simulink library "Valeo_Simulink_Library_EC"  (R2020b)
settings: Solver=ode45  StartTime=0.0  StopTime=10.0  RelTol=1e-3  EnableMultiTasking=on
undefined symbols (not defined in the file): A, B, C, Count_Max, D, InitValue, j, ke, kf, kt, L, Length, MaxIniVal, MaxVal, MinVal, NumBits1, NumBits2, P, p0, Q, R, Simulink_Library, Ts, x0
libraries: $bdroot x9, simulink x4, fixpt_dtprop x4
(part 1 of 4)
Description:
  | This is based on VSL V5.1.0
settings Model: Creator=KROS  LastModifiedBy=mchawa
settings DataIOCC: LimitDataPoints=on  SaveFormat=Array  SignalLoggingSaveFormat=ModelDataLogs  ReturnWorkspaceOutputs=off
settings OptimizationCC: ExpressionDepthLimit=2147483647  LifeSpan=inf
settings DebuggingCC: UnderspecifiedInitializationDetection=Classic  MergeDetectMultiDrivingBlocksExec=none  SolverPrmCheckMsg=warning  MultiTaskDSMMsg=warning  MultiTaskCondExecSysMsg=none  StateNameClashWarn=warning  SFUnexpectedBacktrackingDiag=warning  SFNoUnconditionalDefaultTransitionDiag=warning  SFExecutionAtInitializationDiag=none  ArithmeticOperatorsInVariantConditions=warning
settings HardwareCC: ProdBitPerPointer=32  ProdBitPerSizeT=32  ProdBitPerPtrDiffT=32  ProdLargestAtomicFloat=None  ProdIntDivRoundTo=Undefined  ProdEndianess=Unspecified  ProdWordSize=32  ProdHWDeviceType=32-bit Generic
settings ModelReferenceCC: PropagateSignalLabelsOutOfModel=off
settings SFSimCC: SimUseLocalCustomCode=off  CustomCodeUndefinedFunction=UseInterfaceOnly
settings RTWCC: RTWUseLocalCustomCode=off
settings CodeAppCC: StateflowObjectComments=on
settings GRTTargetCC: TargetLangStandard=C89/C90 (ANSI)
settings ConfigComp: CovMetricSettings=dw  CovSaveCumulativeToWorkspaceVar=on  CovSaveSingleToWorkspaceVar=on  CovExternalEMLEnable=off

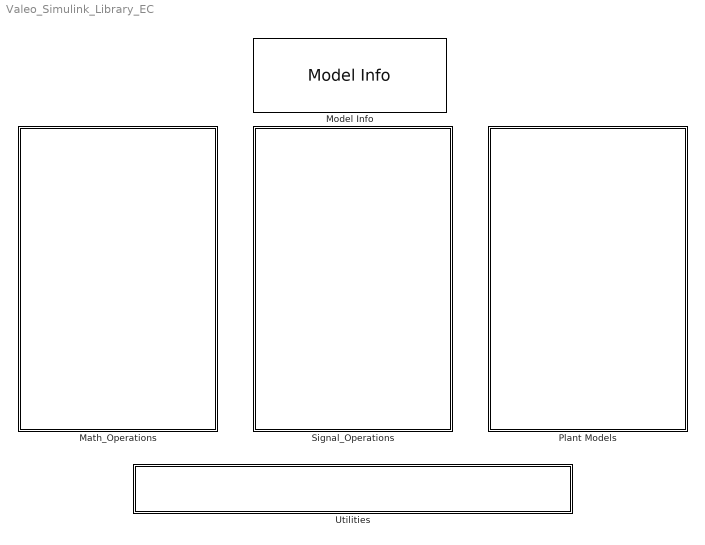
== system Valeo_Simulink_Library_EC ==
  Math_Operations : Subsystem  Description=Math Operations
  Model Info : simulink/Model-Wide Utilities/Model Info  Frame=on  DisplayStringWithTags=|  HorizontalTextAlignment=Left  LeftAlignmentValue=0.02
      | Model Info
      | 
      | Name: %<ModelName>
      | 
      | Description: %<Description>
  Plant Models : Subsystem
  Signal_Operations : Subsystem  Description=Signal Operations
  Utilities : Subsystem  Description=Utilities

== system Valeo_Simulink_Library_EC/Math_Operations ==
  Barycentre : Subsystem  RequirementInfo={} %GIDa_964ea1e7_ae9e_4180_bee1_c2dc4593188a  mask(VSL_Barycentre){}
      mask help:
      | The block 'VSL_Barycentre' calculates the weighted average or centroid of 2 variables 'In1' and 'In2'.
      |
      | Out= In1*Rate+(1-Rate)*In2
      | with 'Rate' value between 0 and 1.
      |
      | In1, In2, Rate et Out must have the same DataType
      | Inputs:
      | - 'In1': fist input for calculation
      | - 'In2': second input for calculation
      | - 'Rate': normalized weight cofficient between 0 and 1
      |
      | Output:
      | - 'Out': centroid value
      mask Help:
      | The block 'VSL_Barycentre' calculates the weighted average or centroid of 2 variables 'In1' and 'In2'.
      | 
      | Out= In1*Rate+(1-Rate)*In2
      | with 'Rate' value between 0 and 1.
      | If 'Rate'>1, 'Rate'=1.
      | If 'Rate'<0, 'Rate'=1.
      | 
      | In1, In2, Rate et Out must have the same DataType
      | Inputs:
      | - 'In1': fist input for calculation
      | - 'In2': second input for calculation
      | - 'Rate': weight cofficient between 0 and 1
      | 
      | Output:
      | - 'Out': weighted average value or centroid
      mask Display:
      | plot([0.3 0.7],[0.4 0.4])
      | plot([0.3 0.5 0.7],[0.4 0.8 0.4])
      | plot([0.3 0.8],[0.4 0.7])
      | plot([0.2 0.7],[0.7 0.4])
      | plot([0.5 0.5],[0.8 0.25])
      | text(0.45,0.59,'G');
      | patch([0.88 0.93 0.94 0.99 0.98 0.94 0.9 0.88], [0.11 0.01 0.01 0.11 0.11 0.026 0.11 0.11], [0 1 0])
  CountdownTimer : Subsystem  Description=CountdownTimer  RequirementInfo={} %GIDa_33143a65_bd33_4657_a3cb_95dcb456cb04  mask(VSL_CountdownTimer){MaxIniVal=MaxIniVal}
      mask prompts: MaxIniVal "Maximum Initial Value:"
      mask help:
      | The 'VSL_CountdownTimer' block performs a countdown from 'IniVal' value (in second), with 'Dec' decrement at each step ('Dec' in second too).
      | A pulse on input 'Strt' launches the countdown.
      | The 'VSL_CountdownTimer' could be reset to 0 if input 'Rst' is set to 1.
      | Reset has higher priority than 'Strt', so nothing happen when 'Rst' is set to 1.
      |
      | The parameter 'MaxIniVal' allows to set the maximum threshold to the initial value.
      |
      | The output 'Out' indicates the countdown status (1 active , 0 inactive) .
      | The counter value 'Val' indicates the remaining time to reach 0 value.
      |
      | The inputs 'Strt' and 'Rst', and the output 'Out' are 'boolean'.
      | 'IniVal', 'Dec', 'Val' are scalars.
      |
      | This block can be used with a variable decrement 'Dec', but the duration ('IniVal') is fixed when it is launched.
      |
      | Inputs:
      | - 'Strt': boolean command with a pulse to launch the countdown
      | - 'Rst': boolean to reset the counter to 0 (all outputs are set to 0 when is equal to 1)
      | - 'IniVal': initial value of duration of the countdown (in second)
      | - 'Dec': sample time (can vary during countdown execution) (in second)
      |
      | Outputs:
      | - 'Out': boolean that indicates the countdown status (1 active , 0 inactive)
      | - 'Val': indicates the remaining time to reach 0 value.
      |
      | Parameter:
      | - 'MaxIniVal': maximum value of the initial value (saturation) (in second)
      settings: AttributesFormatString=MaxIniVal=%<MaxIniVal>
      mask Help:
      | The 'VSL_CountdownTimer' block performs a countdown from 'IniVal' value (in second), with 'Dec' decrement at each step ('Dec' in second too).
      | A pulse on input 'Strt' launches the countdown.
      | The 'CountdownTimer' could be reset to 0 if input 'Rst' is set to 1.
      | Reset has higher priority than 'Strt', so nothing happen when 'Rst' is set to 1.
      | 
      | The parameter 'MaxIniVal' allows to set the maximum threshold to the initial value.
      | 
      | The output 'Out' indicates the countdown status (1 active , 0 inactive) .
      | The counter value 'Val' indicates the remaining time to reach 0 value.
      | 
      | The inputs 'Strt' and 'Rst', and the output 'Out' are 'boolean'.
      | 'IniVal', 'Dec', 'Val' are scalars.
      | 
      | This block can be used with a variable decrement 'Dec', but the duration ('IniVal') is fixed when it is launched.
      | 
      | Inputs:
      | - 'Strt': boolean command with a pulse to launch the countdown
      | - 'Rst': boolean to reset the counter to 0 (all outputs are set to 0 when is equal to 1)
      | - 'IniVal': initial value of duration of the countdown (in second)
      | - 'Dec': sample time (can vary during countdown execution) (in second)
      | 
      | Outputs:
      | - 'Out': boolean that indicates the countdown status (1 active , 0 inactive)
      | - 'Val': indicates the remaining time to reach 0 value.
      | 
      | Parameter:
      | - 'MaxIniVal': maximum value of the initial value (saturation) (in second)
      mask Display:
      | plot(0,0,100,100,[80,70,40,40,30],[20,20,80,20,20])
      | patch(100*[0.88 0.93 0.94 0.99 0.98 0.94 0.9 0.88], 100*[0.11 0.01 0.01 0.11 0.11 0.026 0.11 0.11], [0 1 0])
  Counter : Subsystem  RequirementInfo={} %GIDa_ad99af80_5a44_4606_b9f7_25513ebf5aeb  mask(VSL_Counter){Inc_parm=on, maxFlag=off, Reset_flag=on, InitialFlag=off, MaxCntFlag=off, Cnt_Max=Count_Max}
      mask prompts: Inc_parm "Enable Inc"; maxFlag "Enable MaxFlag"; Reset_flag "Enable Rst"; InitialFlag "Enable InitialVal"; MaxCntFlag "Enable Count_Max"; Cnt_Max "Enter Maximum Value of the Counter"
      mask help:
      | The "VSL_Counter" block increments a counter of the value Inc at each time step if Inc set as a input else counter increment by one when it is activated (Ena = 1). The Cnt output is frozen when the block is deactivated and reset to InitialVal thanks to the "Rst" input (Rst = 1).
      |
      | The Inc and Cnt data are expressed in the same unit, if Inc is expressed in seconds then Cnt is also expressed in seconds.
      |
      | About all inports
      | ------------------------
      | =>  'Inc' is the value of the counter increment per each sample.
      | =>  'Rst' (Boolean) reset the counter (counter start counting from zero if Rst =1).
      | =>  'Ena' (boolean) allows to activate the counter if Ena = 1 else  Deactivate .
      | =>  'InitialVal' can take intial value of the counter for the first sample.
      | =>  'Count_Max'  is a value to count the counter upto this maximum value.
      |
      | About all outports
      | ------------------------
      | => 'Cnt' is counting value of the counter it can update each sample time
      | => 'MaxFlag' (boolean) it is a flag indicates counter reached to Count_Max
      mask init:
      | ValeoSimulinkLibrary.Counter_MaxFlag(gcb);
      | ValeoSimulinkLibrary.Counter_reset(gcb);
      | ValeoSimulinkLibrary.Counter_Inc(gcb);
      | ValeoSimulinkLibrary.Counter_InitialVal(gcb);
      | ValeoSimulinkLibrary.Counter_MaxCount(gcb);
      mask Help:
      | The "VSL_Counter" block can start counting when counter is enable (Ena=1). It can count up to MaxCount, if the Cnt reaches to MaxCount value then Cnt Can be MaxCount value.
      | 
      | User has a flexibility to change the inputs and outputs according to the user need.
      | 
      | Default inputs and outputs
      | ------------------------------
      | 1 > Ena
      | 2 > Cnt
      | 
      | Flexible input and outputs
      | -----------------------------
      | 1 >  Inc
      | 2 > Rst
      | 3 > InitialVal
      | 4 > MaxCount
      | 5 > MaxFlag
      | 
      | 
      | By default counter can increment by one in each sample time. If user wants to increment the counter intentionally with particular value at each sample time user can able to change through the mask input parameter by selecting the check box 'View Inc'.
      | User wants to reset the counters while running the counter then user able to do that through the mask parameter by selecting the check box View Reset.
      | User has flexibility to give initial value through the input parameter from the mask by selecting the 'View InitialVal'. For the First sample InitialVal assign to the Counter. After the sample,counter can increment by Inc in each sample time.
      | 
      | User has a flexibility to give Maximum count as input or mask parameter from the user by selecting the View MaxCount check box. If user selecting the 'View MaxCount' this will be an input parameter. If user can not select the  'View MaxCount' then one text box can popup on the mask window after selecting apply then user need to give the value over there. User cannot enter any value in the edit box then it will give an error message.
      | 
      | User has a flexibility to select 'MaxFlag', From the mask by selecting the 'View MaxFlag' check box. MaxFlag set to one if Cnt reaches to 'MaxCount'
      mask Display:
      | plot([0.1,0.1],[0.1,0.9],[0.08,0.1,0.12],[0.88,0.9,0.88],[0.1,0.9],[0.1,0.1],[0.88,0.9,0.88],[0.08,0.1,0.12],[0.1,0.2,0.2,0.3,0.3,0.4,0.4,0.5,0.5,0.6,0.6,0.7,0.7,0.8,0.8,0.9],[0.1,0.1,0.2,0.2,0.3,0.3,0.4,0.4,0.5,0.5,0.6,0.6,0.7,0.7,0.8,0.8])
      | patch([0.88 0.93 0.94 0.99 0.98 0.94 0.9 0.88], [0.11 0.01 0.01 0.11 0.11 0.026 0.11 0.11], [0 1 0])
  Failure_Counter_Memorisation : Subsystem  Description=This block help to identify failure present in the counter  RequirementInfo={} %GIDa_118737d6_eb19_4cdc_a088_3ba7cacdd147  mask(VSL_Failure Counter memorisation){MAX_CountVal=MaxVal, MIN_CountVal=MinVal, FCM=on, Parameter=Both Min Max}
      mask prompts: MAX_CountVal "Max value of the counter"; MIN_CountVal "Min value of the counter"; FCM "Failure counter memorisation"; Parameter "Select Failure in"
      mask help:
      | Failure counter memorisation used to find failure present in the counter.
      | This counter can work in three different modes.
      |   1> Failure in Maxval.
      |   2> Failure in MinVal.
      |   3> Failure in both min max.
      |
      | "Failure in Maxval" mode used to identify failure present in Maxvalue.
      | "Failure in MinVal" mode used to identify failure present in Minxvalue.
      | "Failure in both min max" mode can identify failure in both min and max values.
      | "Failure memorisation" used to store the first failure until reset the failure memorisation. user can able to select this functionality through the "failure counter memorisation" check box
      mask init:
      | ValeoSimulinkLibrary.Failure_counter_with_memory(gcb);
      | ValeoSimulinkLibrary.FailureCounterM_Inc_Dec_blk_Rvm(gcb);
      mask Help:
      | Failure counter memorisation used to find failure present in the counter.
      | For example User set a maximum value of counter as a MAX_VAL, if counting value of a counter is exceeding "MAX_VAL", then we can say that as failure (it is same for minimum value).
      | If failure happened in the counter then Failure_Memorisation store the first failure, until reset
      | Failure counter Memorisation work in three different modes.
      |   1> Failure in Maxval.
      |   2> Failure in MinVal.
      |   3> Failure in both min max.
      | User have a flexibility to select above three modes from the mask.
      | "Failure Counter memorisation have both increment and decrement counter. "Failure in Maxval" mode acts as an Increment counter. "Failure in MinVal" mode acts as decrement counter.
      | 
      | Functionality
      | -------------
      | Failure counter can increment by INC_Value in each sample, when En_Inc_Counter is enable.
      | Failure counter can decrement by DEC_Value in each sample, when En_Dec_Counter is enable.
      | If User select failure in Maxval mode then Failure_Flag should be one when counting value of counter is greater than Max value else Failure_Flag is zero.
      | If User select failure in Minval mode then Failure_Flag should be one when counting value of counter is less than Min value else Failure_Flag is zero.
      | If User select failure in Both Min Max mode then Failure_Flag should be one when counting value of counter is less than Min value or greater than Max value else Failure_Flag is zero
      | Failure_Memorisation can store first failure until you reset it and after reset Failure_Memorisation will store next failure present in the counter.
      | Failure_Memorisation will be zero when Reset_Failure_Mem is set.
      | Failure_Memorisation Reset functionality can work only when failure is not present in the counter.
      | 
      | 
      | Data types for inports
      | ----------------------------
      | En_Inc_Counter          -> boolean
      | En_Dec_Counter          -> boolean
      | Reset_Failure_Mem       -> boolean
      | DEC_Value               -> Inherit
      | INC_Value               -> Inherit
      | 
      | Data types for Outports
      | ----------------------------
      | Failure_Flag            -> boolean
      | Failure_Memorisation    -> boolean
      mask TypeOptions Parameter: Maxvalue | Minvalue | Both Min Max
      mask Display:
      | plot([0.3,0.3],[0.3,0.9],[0.31,0.3,0.29],[0.88,0.9,0.88])
      | plot([0.3,0.3],[0.3,0.6],[0.3,0.8],[0.3,0.3],[0.78,0.8,0.78],[0.28,0.3,0.32])
      | plot([0.4,0.4,0.5,0.5,0.6,0.6,0.7],[0.3,0.4,0.4,0.5,0.5,0.6,0.6])
      | patch([0.88 0.93 0.94 0.99 0.98 0.94 0.9 0.88], [0.11 0.01 0.01 0.11 0.11 0.026 0.11 0.11], [0 1 0])
      | patch([0.6 0.7],[0.595,0.595],[1 0 0])
  SecureDiv : Subsystem  Description=SecureDiv  RequirementInfo={} %GIDa_e566a2ca_2479_49c1_9747_e44ec0414da5  mask(VSL_SecureDiv){SatAbsDen=0.01, SatMinDiv=-3276.8, SatMaxDiv=3276.7, Nan_alt_value=0}
      mask prompts: SatAbsDen "Absolute minimum value of denominator (value > 0)"; SatMinDiv "Minimum division output saturation value"; SatMaxDiv "Maximum division output saturation value"; Nan_alt_value "Nan recovery value"
      mask help:
      | The aim is to divide numerator 'Num' by denominator 'Den', and saturate the output between parameters: 'SatMin' and 'SatMax'.
      | To avoid division by 0, a parameter shall be filled for absolute minimum value of denominator 'Den'.
      |
      | Inputs:
      | - 'Num': numerator
      | - 'Den': denominator
      |
      | Output:
      | - 'Out': result of the secure division
      |
      | Block parameters:
      | - 'SatAbsDen': Absolute minimum value of denominator (value > 0)
      |     If abs('Den')<'SatAbsDen' then Output=Num/SatAbsDen
      | - 'SatMinDiv': Minimum division output saturation value
      | - 'SatMaxDiv': Maximum division output saturation value
      | - 'Nan_alt_value': Nan recovery value
      mask init:
      | if SatAbsDen == 0
      |        error(' !! The absolute minimum value of denominator must be different from zero !!');
      | 
      | end;    
      |     
      | ListLine = find_system(gcb,'FollowLinks','on','findall','on','LookUnderMasks','all','SearchDepth',1,'Type','line');
      | ListBLKO = find_system(gcb,'FollowLinks','on','SearchDepth',1,'LookUnderMasks','all','BlockType', 'Outport');
      | 
      | BFlagSat = find_system(gcb,'FollowLinks','on','SearchDepth',1,'LookUnderMasks','all','BlockType', 'Outport','Name','FlagSat');
      | BTFlagSat = find_system(gcb,'FollowLinks','on','SearchDepth',1,'LookUnderMasks','all','BlockType', 'Terminator','Name','FlagSat');
      | 
      | if SatMaxDiv == Inf
      |     SatMaxDiv=3.0E38;
      | end;
      | 
      | if SatMaxDiv == -Inf
      |     SatMaxDiv=-3.0E38;
      | end;
      | 
      | if SatMinDiv == -Inf
      |     SatMinDiv=-3.0E38;
      | end;
      | 
      | if SatMinDiv == Inf
      |     SatMinDiv=3.0E38;
      | end;
      settings: AttributesFormatString=|
      | Abs. Sat. of Den. : %<SatAbsDen>
      | Min. Sat. of Out : %<SatMinDiv>
      | Max. Sat. of Out : %<SatMaxDiv>
      | Nan_alt_value: %<Nan_alt_value>
      mask Help:
      | The aim is to divide numerator 'Num' by denominator 'Den', and saturate the output between parameters: 'SatMin' and 'SatMax'.
      | To avoid division by 0, a parameter shall be filled for absolute minimum value of denominator 'Den'.
      | 
      | Inputs:
      | - 'Num': numerator
      | - 'Den': denominator
      | 
      | Output:
      | - 'Out': result of the secure division
      | 
      | Block parameters:
      | - 'SatAbsDen': Absolute minimum value of denominator (value > 0)
      |     If abs('Den')<'SatAbsDen' then Output=Num/SatAbsDen
      | - 'SatMinDiv': Minimum division output saturation value
      | - 'SatMaxDiv': Maximum division output saturation value
      | - 'Nan_alt_value': Nan recovery value
      |     If 'Num'/'Den'= 0/0--> 'Out'='Nan_alt_value'
      mask Display:
      | disp('Num\n---------\nDen')
      | 
      | 
      | patch([0.88 0.93 0.94 0.99 0.98 0.94 0.9 0.88], [0.11 0.01 0.01 0.11 0.11 0.026 0.11 0.11], [0 1 0])
  VSL_DynamicSecureDivision_EC_Blk : Subsystem  Description=the block performs a Secure Division with dynamic values for P_inf, N_inf and Nan  RequirementInfo={} %GIDa_6d541c2f_44eb_458a_83e9_371ff57090ab  TreatAsAtomicUnit=on  RTWFcnName=ClarkTransformation  mask(Dynamic Secure Division){ZeroBand_Num=eps, ZeroBand_Den=eps}
      mask prompts: ZeroBand_Num "ZeroBand_Num : Numerator has to be greater than ZeroBand_Num to be considered as non-zero"; ZeroBand_Den "ZeroBand_Den : denominator has to be greater than ZeroBand_Den to be considered as non-zero"
      mask help:
      | Dynamic Secure Division block to protect aginst division by zero
      | and to dynamiclly assign values to the output in case of P_inf, N_inf or Nan
      | eps is used as default value in case of floating data types ( insted of zero )
      | to handle float equality as eps is the min value matlab can recognize
      settings: RTWFcnNameOpts=User specified
      mask Display:
      | plot(0,0,100,100)
      | patch(100*[0.88 0.93 0.94 0.99 0.98 0.94 0.9 0.88], 100*[0.11 0.01 0.01 0.11 0.11 0.026 0.11 0.11], [0 1 0])
      | disp(['Dynamic \n' char(10) 'Secure Division']);

== system Valeo_Simulink_Library_EC/Plant Models ==
  Actuators : Subsystem
  Sensors : Subsystem

== system Valeo_Simulink_Library_EC/Signal_Operations ==
  DKLowPassFilter_FixPt : Subsystem  Description=DKLowPassFilter_FixPt  RequirementInfo={} %GIDa_d4aeea3d_863f_419d_a2bc_912ff2a67fc8  TreatAsAtomicUnit=on  mask(VSL_DLowPassFilter_FixPt){}
      mask help:
      | First order low pass filter with a normalized cutoff frequency 'K' between 0 and 1:
      | This bloc must be used in fixed point models ( an additionnal calculation is added to force the output convergence)
      |
      | K, In, Init, And Out must have the same data Type
      |
      | Out(n) =  K * (In(n) - Out(n-1))   + Out(n-1)
      | with : K = cutoff frequency(Hz, radians)/ sampling frequency(Hz,radians)
      | K=1 : no filter => Out = In
      | K=0 : one step delay => Out(n)=Out(n-1)
      | At initialization or when Rst=1: Out = Init
      |
      | Remark to use this filter:
      | This filter can be with variable normalized cutoff frequency 'K'.
      mask Help:
      | First order low pass filter with a normalized cutoff frequency 'K' between 0 and 1:
      | This bloc must be used in fixed point models ( an additionnal calculation is added to force the output convergence)
      | K, In, Init, And Out must have the same data Type
      | 
      | Out(n) =  K * (In(n) - Out(n-1))   + Out(n-1)
      | with : K = cutoff frequency(Hz, radians)/ sampling frequency(Hz,radians)
      | K=1 : no filter => Out = In
      | K=0 : one step delay => Out(n)=Out(n-1)
      | At initialization or when Rst=1: Out = Init
      | 
      | Remark to use this filter:
      | This filter can be with variable normalized cutoff frequency 'K'.
      mask Display:
      | plot(0,0,100,100, [10,13,13,16,16,18],[4,4,15,15,4,4],  [73,75,73,75,29,29,31,29,28], [17,20,23,20,20,88,86,88,86],  [29,75], [70,70],  [29,30,32,35,40,46,52,62,75], [20,25,33,43,55,63,66,67,67],  [55,55],[40,51],[55,60],[45,51],[56,60],[46,40] )
      | patch(100*[0.88 0.93 0.94 0.99 0.98 0.94 0.9 0.88], 100*[0.11 0.01 0.01 0.11 0.11 0.026 0.11 0.11], [0 1 0])
  DKLowPassFilter_Float : Subsystem  Description=DKLowPassFilter_Float  RequirementInfo={} %GIDa_90f8789e_b237_41a4_8feb_99f737a5412d  TreatAsAtomicUnit=on  mask(VSL_DLowPassFilter_Float){}
      mask help:
      | First order low pass filter with a normalized cutoff frequency 'K' between 0 and 1:
      | This bloc must be used only in float models
      |
      | Out(n) =  K * (In(n) - Out(n-1))   + Out(n-1)
      | with : K = cutoff frequency(Hz, radians)/ sampling frequency(Hz,radians)
      | K=1 : no filter => Out = In
      | K=0 : one step delay => Out(n)=Out(n-1)
      | At initialization or when Rst=1: Out = Init
      |
      | Remark to use this filter:
      | This filter can be with variable normalized cutoff frequency 'K'.
      mask Help:
      | First order low pass filter with a normalized cutoff frequency 'K' between 0 and 1:
      | This bloc must be used only in float models
      | 
      | Out(n) =  K * (In(n) - Out(n-1))   + Out(n-1)
      | with : K = cutoff frequency(Hz, radians)/ sampling frequency(Hz,radians)
      | K=1 : no filter => Out = In
      | K=0 : one step delay => Out(n)=Out(n-1)
      | At initialization or when Rst=1: Out = Init
      | 
      | Remark to use this filter:
      | This filter can be with variable normalized cutoff frequency 'K'.
      mask Display:
      | plot(0,0,100,100, [10,13,13,16,16,18],[4,4,15,15,4,4],  [73,75,73,75,29,29,31,29,28], [17,20,23,20,20,88,86,88,86],  [29,75], [70,70],  [29,30,32,35,40,46,52,62,75], [20,25,33,43,55,63,66,67,67],  [55,55],[40,51],[55,60],[45,51],[56,60],[46,40] )
      | patch(100*[0.88 0.93 0.94 0.99 0.98 0.94 0.9 0.88], 100*[0.11 0.01 0.01 0.11 0.11 0.026 0.11 0.11], [0 1 0])
  Debouncing_Blk : Subsystem  Description=Debouncing Block  RequirementInfo={} %GIDa_c4ebdc17_05b4_47bc_b09c_4c6456a96248  mask(VSL_DebouncingBlock){Rst_Flag=off, Cnt_Flag=off}
      mask prompts: Rst_Flag "External Reset"; Cnt_Flag "External Counter"
      mask help:
      | Debouncing algorithm is used to filter out transient Signals that do not present a true change of state.
      |
      | DESCRIPTION
      | -----------------
      |
      | IN               | OUT Prev         | Counter
      | ------------------------------------------------
      | FALSE        |     TRUE            |  Counter + INC
      | FALSE        |     FALSE           |  Reset Counter
      | TRUE         |     TRUE            |  Reset Counter
      | TRUE         |     FALSE           |  Counter + INC
      |
      | Reset |Prev OUT |Counter         |OUT       |Counter
      | -----------------------------------------------------
      | 0     |TRUE     |> Turn_Off THR  | FALSE    | 0
      | 0     |FALSE    |> Turn_ON THR   | TRUE     | 0
      | 0     | -           |Else                | Prev OUT | Counter
      | 1     | -           |-                   | Init     | 0
      mask init:
      | ValeoSimulinkLibrary.Debouncing_ConfigRst_Cnt(gcb);
      mask Display:
      | plot(0,0,100,100,[14 23 23 24 24 25 25 26 26 27 27 28 28 30 30 70 70 72 72 74 74 76 76 77 77 78 78 79 79 90],[60 60 80 80 60 60 80 80 60 60 80 80 60 60 80 80 60 60 80 80 60 60 80 80 60 60 80 80 60 60],[14 35 35 83 83 90], [30 30 50 50 30 30])
      | patch(100*[0.88 0.93 0.94 0.99 0.98 0.94 0.9 0.88], 100*[0.11 0.01 0.01 0.11 0.11 0.026 0.11 0.11], [0 1 0])
  DetectSat : Subsystem  Description=DetectSat  RequirementInfo={} %GIDa_3ae17530_8fb8_4519_b0fd_dc2823ce1693  mask(VSL_DetectSat){FlagHitMax=off, FlagHitMin=off, FlagOut=on, FlagRevThr=off, EnableRevThreshold=No, LibType=Simulink_Library}
      mask prompts: FlagHitMax "View HitMax"; FlagHitMin "View HitMin"; FlagOut "View Output"; FlagRevThr "View Reversed Thresholds Flag"; EnableRevThreshold "Allow Reversed Polarity (If SatMax < SatMin )"; LibType "Library Type"
      mask help:
      | This block saturates the input between 2 values 'SatMax' and 'SatMin' and raises flag that saturation occurs if input reaches either maximum value(HitMax) or minimum value(HitMin).
      |
      | If the input is less than 'SatMin', Output = 'SatMin' and HitMin = 1
      | Else If the input is greater than 'SatMax', Ouput = 'SatMax' and HitMax=1
      | Else Output is equal to input also 'HitMin' and 'Hitmax' will be equal to 0.
      |
      | If reversed polarity is allowed,then 'SatMax' = Max('SatMax','SatMin') and 'SatMin' = Min('SatMax','SatMin')
      |
      | Parameters 'View Output','View HitMin','View Reversed Thresholds Flag' and 'View HitMax' are added to terminate or view 'Out', 'HitMax', 'ReversedThr' and 'HitMin'.
      mask init:
      | ValeoSimulinkLibrary.DetectSat_ReversedPolarity(gcb);
      | 
      | ValeoSimulinkLibrary.DetectSat_NormalMode(gcb);
      | 
      | %SMBDP-REQ-0017(0),SMBDP-REQ-0012(0)
      | ValeoSimulinkLibrary.DetectSat_View_Terminate(gcb);
      | 
      | ValeoSimulinkLibrary.DetectSat_SortOutports(gcb);
      mask Help:
      | Block Functionality:<br>
      | This block saturates the input between 2 values 'SatMax' and 'SatMin' and raises flag that saturation occurs if input reaches either maximum value(HitMax) or minimum value(HitMin).
      | <br>
      | Block Interfaces and constrains:<br>
      | 	Output, saturation maximum and minimum thresholds imposed to have the same datatype as Input
      | 	Saturation maximum and minimum thresholds could be dynamic, so it's better to allow reversed threshold mode
      |     if 'SatMax' could hold value less than 'SatMin'.
      | 	User can display or hide any of the block outputs based on the parameters 'View Output','View HitMin','View Reversed Thresholds Flag' and 'View HitMax'.
      | <br>
      | Block Logic:<br>
      | 	If the input is less than 'SatMin', Output = 'SatMin' and HitMin = 1
      | 	Else If the input is greater than 'SatMax', Ouput = 'SatMax' and HitMax=1
      | 	Else Output is equal to input also 'HitMin' and 'Hitmax' will be equal to 0.
      |    User could allow reversed polarity mode if SatMax could take value less than SatMin
      |    In this mode: 'SatMax' = Max('SatMax','SatMin') and 'SatMin' = Min('SatMax','SatMin'), also
      |     'ReversedThr' output is equal to 1 only when 'SatMax' < 'SatMin'.
      | <br>
      mask TypeOptions EnableRevThreshold: Yes | No
      mask Display:
      | plot([0.2 0.8],[0.5 0.5],[0.5 0.5],[0.05 0.95],[0.1 0.4 0.6 0.9],[0.05 0.05 0.95 0.95])
      | patch([0.88 0.93 0.94 0.99 0.98 0.94 0.9 0.88], [0.11 0.01 0.01 0.11 0.11 0.026 0.11 0.11], [0 1 0])
  FallingEdge : Subsystem  Description=FallingEdge  RequirementInfo={} %GIDa_22203cf7_274b_4877_a67f_94181d6e1736  mask(VSL_FallingEdge){INIT=0}
      mask prompts: INIT "Activation at Initialization"
      mask help:
      | - Falling edge detection for a logic signal.
      |
      | - When a falling edge on the input signal is detected, the output switches to 1 during one computation period.
      |
      | - Activation at initialization parameter (AAI) is used to activate the block at the initialization :
      |
      | at t=0 :
      |
      |   AAI |  IN  | OUT
      | -------------------
      |   0   |  0   | 0
      |   0   |  1   | 0
      |   1   |  0   | 1
      |   1   |  1   | 0
      mask init:
      | if strcmpi(INIT,'0')
      | 	Init=0;
      | else
      | 	Init=1;
      | end
      mask Help:
      | Activation at initialization parameter (AAI) is used to activate the block at the initialization :
      | 
      | at t=0 :
      | 
      |   AAI |  IN  | OUT
      | -------------------
      |   0   |  0   | 0
      |   0   |  1   | 0
      |   1   |  0   | 1
      |   1   |  1   | 0
      mask TypeOptions INIT: 0 | 1
      mask Display:
      | plot(0,0,100,100, [20 50 50 80], [90 90 10 10], [40 50 60], [55 45 55] )
      | patch(100*[0.88 0.93 0.94 0.99 0.98 0.94 0.9 0.88], 100*[0.11 0.01 0.01 0.11 0.11 0.026 0.11 0.11], [0 1 0])
  KalmanFilter_single : Subsystem  RequirementInfo={} %GIDa_274cb745_29bd_4c47_bb05_149739b18e29  TreatAsAtomicUnit=on  SystemSampleTime=Ts  mask(VSL_KalmanFilter_single){A=A, B=B, C=C, D=D, x0=x0, p0=p0, Q=Q, R=R, Ts=Ts}
      mask prompts: x0 "Initial states x[0]:"; p0 "Initial error Covariance p[0]:"; Ts "Sample Time"
      mask help: Kalman filter is an optimal filter used to filter out stochastic noise imposed on signals, by incorporating linear process model for state prediction and optimally calculating observer gain to minimize the mean square error of prediction covariance.
      mask Help: Kalman filter is an optimal filter used to filter out stochastic noise imposed on signals, by incorporating linear process model for state prediction and optimally calculating observer gain to minimize the mean square error of prediction covariance.
      mask Display:
      | plot(0,0,100,100)
      | patch(100*[0.88 0.93 0.94 0.99 0.98 0.94 0.9 0.88], 100*[0.11 0.01 0.01 0.11 0.11 0.026 0.11 0.11], [0 1 0])
  Mem : Subsystem  Description=Mem  RequirementInfo={} %GIDa_258f40ab_f7f5_4bf3_807b_00fdb725a09e  TreatAsAtomicUnit=on  mask(VSL_Mem){InitVal=InitValue}
      mask prompts: InitVal "Initial value (of the held output)"
      mask help:
      | The block 'Mem' allow to save and hold a signal value 'In' when 'Hld' is set to 1.
      |
      | Output "Out"  :
      | - is equal to 'In' if 'Hld'=0
      | - is equal to previous 'Out' value if 'Hld'=1
      mask Help:
      | The block 'Mem' allow to save and hold a signal value 'In' when 'Hld' is set to 1.
      | <br><br>
      | Inputs are : input signal 'In' and block command 'Hld' (Boolean).
      | <br><br>
      | Output "Out" :<br>
      | - is equal to 'In' if 'Hld'=0<br>
      | - is equal to previous 'Out' value if 'Hld'=1
      | <br><br>
      | 'In' and 'Out' have the same datatype.
      | <br><br>
      | Block is working if sample time is between: 1ms and 2s.
      mask Display:
      | plot([0.2,0.85,0.85,0.2,0.2],[0.1,0.1,0.9,0.9,0.5],[0.17,0.2,0.23],[0.53,0.5,0.53],[0.15,0.18,0.18,0.22,0.22,0.25],[0.2,0.2,0.35,0.35,0.2,0.2])
      | patch([0.88 0.93 0.94 0.99 0.98 0.94 0.9 0.88], [0.11 0.01 0.01 0.11 0.11 0.026 0.11 0.11], [0 1 0])
  NegHys : Subsystem  Description=NegHys  RequirementInfo={} %GIDa_82e62a24_d7f3_4584_a92d_6951279c234b  TreatAsAtomicUnit=on  mask(VSL_NegHys){}
      mask help:
      | * This block allows to generate a Negative hysteresis signal.
      | * The input signal is compared with the "High" and "Low" inputs.
      | * 'High' threshold and 'Low' threshold could be variable signals
      |
      | * 'In', 'High' and 'Low' must have the same data type
      | * 'Out' : The output signal is defined as a boolean
      |
      | Operating case:
      |
      | 	- In <= Low  then  Out = 1;
      | 	- In > Low and In >= High   then Out = 0;
      | 	- In > Low  and In < High then Out = Old_Value;
      |
      | Note : If High <= Low the same algorithm is applied.
      mask Help:
      | * This block allows to generate a Negative hysteresis signal.
      | * The input signal is compared with the "High" and "Low" inputs.
      | * 'High' threshold and 'Low' threshold could be variable signals
      | 
      | * 'In', 'High' and 'Low' must have the same data type
      | * 'Out' : The output signal is defined as a boolean
      | 
      | Operating case:
      | 
      | 	- In <= Low  then  Out = 1;
      | 	- In > Low and In >= High   then Out = 0;
      | 	- In > Low  and In < High then Out = Old_Value;
      | 
      | Note : If High <= Low the same algorithm is applied.
      mask Display:
      | plot([0.1,0.7,0.7,0.9],[0.9,0.9,0.1,0.1],[0.3,0.3,0.7],[0.9,0.1,0.1],[0.25,0.3,0.35],[0.50,0.57,0.50],[0.65,0.7,0.75],[0.5,0.43,0.5])
      | patch([0.88 0.93 0.94 0.99 0.98 0.94 0.9 0.88], [0.11 0.01 0.01 0.11 0.11 0.026 0.11 0.11], [0 1 0])
  PosHys : Subsystem  Description=PosHys  RequirementInfo={} %GIDa_c2ad47c6_50e1_43df_97f1_d9465da51641  TreatAsAtomicUnit=on  mask(VSL_PosHys){}
      mask help:
      | * This block allows to generate a Positive hysteresis signal.
      | * The input signal is compared with the "High" and "Low" inputs.
      | * 'High' threshold and 'Low' threshold could be variable signals
      |
      | * 'In', 'High' and 'Low' must have the same data type
      | * 'Out' : The output signal is defined as a boolean
      |
      | Operating case:
      |
      | 	- In <= Low  then  Out = 0;
      | 	- In > Low and In >= High   then Out = 1;
      | 	- In > Low  and In < High then Out = Old_Value;
      |
      | Note : If High <= Low the same algorithm is applied.
      mask Help:
      | * This block allows to generate a Positive hysteresis signal.
      | * The input signal is compared with the "High" and "Low" inputs.
      | * 'High' threshold and 'Low' threshold could be variable signals
      | 
      | * 'In', 'High' and 'Low' must have the same data type
      | * 'Out' : The output signal is defined as a boolean
      | 
      | Operating case:
      | 
      | 	- In <= Low  then  Out = 0;
      | 	- In > Low and In >= High   then Out = 1;
      | 	- In > Low  and In < High then Out = Old_Value;
      | 
      | Note : If High <= Low the same algorithm is applied.
      mask Display:
      | plot([0.1,0.7,0.7,0.9],[0.1,0.1,0.9,0.9],[0.3,0.3,0.7],[0.1,0.9,0.9],[0.25,0.3,0.35],[0.5,0.43,0.5],[0.65,0.7,0.75],[0.50,0.57,0.50])
      | patch([0.88 0.93 0.94 0.99 0.98 0.94 0.9 0.88], [0.11 0.01 0.01 0.11 0.11 0.026 0.11 0.11], [0 1 0])
  RisingEdge : Subsystem  Description=RisingEdge  RequirementInfo={} %GIDa_2e5d1dc6_de22_4421_94d1_5b2754cd9bec  mask(VSL_RisingEdge){INIT=0}
      mask prompts: INIT "Activation at Initialization"
      mask help:
      | - Rising edge detection for a logic signal.
      |
      | - When a rising edge on the input signal is detected, the output switches to 1 for only one computation period.
      |
      | - Activation at initialization parameter (AAI) is used to activate the block at the initialization :
      |
      | at t=0 :
      |
      |   AAI |  IN  | OUT
      | -------------------
      |   0   |  0   | 0
      |   0   |  1   | 0
      |   1   |  0   | 0
      |   1   |  1   | 1
      mask init:
      | if strcmpi(INIT,'0')
      | 	Init=0;
      | else
      | 	Init=1;
      | end
      mask Help:
      | Block Functionality:
      | 
      | If input is equal to zero and it changes its state to be one, then the output should be one for only one step.
      | 
      | Block Interfaces and constrains:
      | 
      |  Input and Output are booleans.
      | 
      | Activation at initialization parameter (AAI)is used to activate the block at the initialization :
      | 
      | at t=0 :
      | 
      |   AAI |  IN  | OUT
      | -------------------
      |   0   |  0   | 0
      |   0   |  1   | 0
      |   1   |  0   | 0
      |   1   |  1   | 1
      mask TypeOptions INIT: 0 | 1
      mask Display:
      | plot(0,0,100,100, [20 50 50 80], [10 10 90 90], [40 50 60], [45 55 45] )
      | patch(100*[0.88 0.93 0.94 0.99 0.98 0.94 0.9 0.88], 100*[0.11 0.01 0.01 0.11 0.11 0.026 0.11 0.11], [0 1 0])
  SlidingAverageFiltrer : Subsystem  Description=Sliding average Filter computes the moving average of the input signal along each channel, independently over time  RequirementInfo={} %GIDa_407742ea_d191_4a40_a464_a74cc348d730  mask(VSL_SlidingAverageFilter){WindowLength=4, InputTypeFlag=off}
      mask prompts: WindowLength "Window Length"; InputTypeFlag "Input Type is 32 bits ?"
      mask help:
      | Sliding average Filter computes the moving average of the input signal along each channel, independently over time.
      | The output for each input sample is the statistic over the window of the current sample and the Len - 1 previous samples.
      | In the first-time step, to compute the first Len - 1 outputs, the algorithm fills the window with zeros.
      |
      |  Window length  Length of sliding window
      |     4 (default) | positive scalar integer
      |
      |  Input Type is 32 bits? : Flag to specify if the input Type is an 32 bits or not
      | true  The input is a 32 bits data (uint32, int2, fixdt(0, 32, ..)
      | false  The input d is different from 32 bits data (uint32, int2, fixdt(0, 32, ..)
      |
      | Effect of Window Length
      | - For data that does not change rapidly, use a long window to get a smoother statistic.
      | - For data that changes fast, use a smaller window.
      |
      | Use the Help to get an example
      mask init:
      | if WindowLength == 0
      |        error(' !! The window Length must be different from zero !!');
      | end;
      | 
      | ValeoSimulinkLibrary.SAF_TypeProp(gcb);
      mask Help:
      | The output for each input sample is the statistic over the window of the current sample and the Len - 1 previous samples. In the first-time step, to compute the first Len - 1 outputs when the window does not have enough data yet, the algorithm fills the window with zeros. In the subsequent time steps, to fill the window, the algorithm uses samples from the previous data frame. The moving statistic algorithms have a state and remember the previous data.
      | 
      | An example with Window Length = 4:
      | Moving Average filter takes the current and previous 3 samples of input and calculates the average. This operation is represented as bellow:
      | Window fills with zeros until window length of 4 is reached
      | 
      | Current   |  Input | Sliding Average Filter compute |	 Output
      | Sample
      | 
      | n=0       | 2        | = (2 + 0 + 0 + 0) / 4               |0.5
      | n=1       | 4        | = (2 + 4 + 0 + 0) / 4               |1.5
      | n=2       | 6		 | = (2 + 4 + 6 + 0) / 4               |3
      | n=3       | 8		 | = (2 + 4 + 6 + 8) / 4               |5
      | n=4       | 9		 | = (4 + 6 + 8 + 9) / 4               |6.75
      mask Display:
      | plot(0,0,100,100)
      | patch(100*[0.88 0.93 0.94 0.99 0.98 0.94 0.9 0.88], 100*[0.11 0.01 0.01 0.11 0.11 0.026 0.11 0.11], [0 1 0])
      | disp(['Sliding' char(10) 'Average Filter']);
  TurnOffDelay : Subsystem  Description=TurnOffDelay  RequirementInfo={} %GIDa_c135e972_991e_4c6d_bd3c_66f8d1db9c74  TreatAsAtomicUnit=on  mask(VSL_TurnOffDelay){}
      mask help:
      | This block aim is to delay with 'Tdly' the desactivation of a signal 'In'.
      |
      |
      | Inputs:
      | - 'In': signal to treat (boolean)
      | - 'Tdly': duration of delay
      | - 'Te': sample time
      |
      | - 'Tdly' and 'Te' must have the same data type
      | - Te must be >= 'solver sample time' and >0
      |
      | Output:
      | - 'Out': signal with delay on activation (boolean)
      |
      | When 'Tdly' is not a multiple of 'Te', the delay will be the multiple round value (and superior to 'Te').
      mask Help:
      | This block aim is to delay with 'Tdly' the desactivation of a signal 'In'.
      | This block can generate one step delay in some case when using single propagation
      | 
      | Inputs:
      | - 'In': signal to treat (boolean)
      | - 'Tdly': duration of delay
      | - 'Te': sample time
      | 
      | - 'Tdly' and 'Te' must have the same data type
      | - Te must be >= 'solver sample time' and >0
      | 
      | Output:
      | - 'Out': signal with delay on activation (boolean)
      | 
      | When 'Tdly' is not a multiple of 'Te', the delay will be the multiple round value (and superior to 'Te').
      mask Display:
      | plot([0.1 0.65 0.65 0.9],[0.9 0.9 0.25 0.25]);
      | plot([0.1 0.35 0.35 0.9],[0.75 0.75 0.1 0.1]);
      | 
      | %All
      | plot([0.35 0.65],[0.5 0.5]);
      | text(0.43,0.55,'Tdly');
      | plot([0.4 0.35 0.4],[0.48 0.5 0.52]);
      | plot([0.6 0.65 0.6],[0.48 0.5 0.52]);
      | patch([0.88 0.93 0.94 0.99 0.98 0.94 0.9 0.88], [0.11 0.01 0.01 0.11 0.11 0.026 0.11 0.11], [0 1 0]);
  TurnOnDelay : Subsystem  Description=TurnOnDelay  RequirementInfo={} %GIDa_45d05c0c_a964_4d3b_ba9a_6635738b8bcd  TreatAsAtomicUnit=on  mask(VSL_TurnOnDelay){}
      mask help:
      | This block aim is to delay with 'Tdly' the activation of a signal 'In'.
      |
      |
      | Inputs:
      | - 'In': signal to treat (boolean)
      | - 'Tdly': duration of delay
      | - 'Te': sample time
      |
      | - 'Tdly' and 'Te' must have the same data type
      | - Te must be >= 'solver sample time' and >0.
      |
      | Output:
      | - 'Out': signal with delay on activation (boolean)
      |
      | When 'Tdly' is not a multiple of 'Te', the delay will be the multiple round value (and superior to 'Te').
      mask Help:
      | This block aim is to delay with 'Tdly' the activation of a signal 'In'.
      | 
      | This block can generate one step delay in some case when using single propagation
      | Inputs:
      | - 'In': signal to treat (boolean)
      | - 'Tdly': duration of delay
      | - 'Te': sample time
      | 
      | - 'Tdly' and 'Te' must have the same data type
      | - Te must be >= 'solver sample time' and >0
      | 
      | Output:
      | - 'Out': signal with delay on activation (boolean)
      | 
      | When 'Tdly' is not a multiple of 'Te', the delay will be the multiple round value (and superior to 'Te').
      mask Display:
      | plot([0.9 0.65 0.65 0.1],[0.75 0.75 0.1 0.1]);
      | plot([0.9 0.35 0.35 0.1],[0.9 0.9 0.25 0.25]);
      | 
      | %All
      | plot([0.35 0.65],[0.5 0.5]);
      | text(0.43,0.55,'Tdly');
      | plot([0.4 0.35 0.4],[0.48 0.5 0.52]);
      | plot([0.6 0.65 0.6],[0.48 0.5 0.52]);
      | patch([0.88 0.93 0.94 0.99 0.98 0.94 0.9 0.88], [0.11 0.01 0.01 0.11 0.11 0.026 0.11 0.11], [0 1 0]);
  VSL_ClarkTransformation_EC_Blk : Subsystem  Description=This Block transforms the a-b-c quantities to alpha-beta quantities (stationary frame)  RequirementInfo={} %GIDa_d73c7d72_ab0d_420b_9b1a_f28e9ca9498a  TreatAsAtomicUnit=on  RTWFcnName=ClarkTransformation  mask(Clark Transformation){}
      mask help: Clark Transformation is a linear transformation from abc to apha-beta
      settings: RTWFcnNameOpts=User specified
      mask Display:
      | plot(0,0,100,100)
      | patch(100*[0.88 0.93 0.94 0.99 0.98 0.94 0.9 0.88], 100*[0.11 0.01 0.01 0.11 0.11 0.026 0.11 0.11], [0 1 0])
      | disp(['Clark' char(10) 'Transformation']);
  VSL_InverseClarkTransformation_EC_Blk : Subsystem  Description=This Block transforms the alpha-beta quantities (stationary frame) to a-b-c quantities  RequirementInfo={} %GIDa_b9ed04c0_6072_41c9_a001_61df739c080f  TreatAsAtomicUnit=on  RTWFcnName=ClarkTransformation  mask(Inverse Clark Transfrom){}
      mask help: this block is transforming alpha-beta axis to abc axis
      settings: RTWFcnNameOpts=User specified
      mask Display:
      | plot(0,0,100,100)
      | patch(100*[0.88 0.93 0.94 0.99 0.98 0.94 0.9 0.88], 100*[0.11 0.01 0.01 0.11 0.11 0.026 0.11 0.11], [0 1 0])
      | disp(['Inverse Clark' char(10) 'Transformation']);
  VSL_InverseParkTransformation_EC_Blk : Subsystem  Description=This Block is transforming dq axies into alpha-beta  RequirementInfo={} %GIDa_647746a6_9a4d_4075_938c_92d76514c259  TreatAsAtomicUnit=on  RTWFcnName=Park_Transformation  mask(Inverse Park Transformation){}
      mask help: Inverse Park Transformation is a linear transformation that transforms dq axies into alpha beta ones .
      settings: RTWFcnNameOpts=User specified
      mask Display:
      | plot(0,0,100,100)
      | patch(100*[0.88 0.93 0.94 0.99 0.98 0.94 0.9 0.88], 100*[0.11 0.01 0.01 0.11 0.11 0.026 0.11 0.11], [0 1 0])
      | disp(['Inverse Park' char(10) 'Transformation']);
  VSL_ParkTransformation_Blk : Subsystem  Description=Park Transformation  RequirementInfo={} %GIDa_f3ced52f_47f3_4b7a_b6d3_566be3aa0ab2  TreatAsAtomicUnit=on  RTWFcnName=Park_Transformation  mask(Park Transfromation){}
      mask help: This Block is transforming alpha-beta axises into dq axies, d is aligned with Phase A
      settings: RTWFcnNameOpts=User specified
      mask Display:
      | plot(0,0,100,100)
      | patch(100*[0.88 0.93 0.94 0.99 0.98 0.94 0.9 0.88], 100*[0.11 0.01 0.01 0.11 0.11 0.026 0.11 0.11], [0 1 0])
      | disp(['Park' char(10) 'Transformation']);
  VSL_SpaceVectorModulation_EC_Blk : Subsystem  Description=this block impelements Space Vector modulation with rotating Active zero vector  RequirementInfo={} %GIDa_763e7ff4_86de_426e_a38f_c108c2d4fb2a  mask(Space Vector Modulation){}
      mask help:
      | This block implements SVM
      | the inputs A, B, C are the refrance volatge of the three phases
      | Da_U, Db_U and Dc_U are duty cycles for upper switches.
      | Da_L, Db_L and Dc_L are duty cycles for Lower switches.
      mask Display:
      | plot(0,0,100,100)
      | patch(100*[0.88 0.93 0.94 0.99 0.98 0.94 0.9 0.88], 100*[0.11 0.01 0.01 0.11 0.11 0.026 0.11 0.11], [0 1 0])
      | disp(['Space Vector \n' char(10) 'Modulation']);

== system Valeo_Simulink_Library_EC/Utilities ==
  EventToVar : Subsystem  Description=EventToVar  RequirementInfo={} %GIDa_4ababea4_0407_4080_8ed3_305b044ebc1f  mask(VSL_EventToVar){}
      mask help:
      | Transform an event into a boolean variable data.
      | - The block transforms every event into a pulse signal with pulse width equal to adopted step size.
      | - Could be used for validation purpose.
      mask Help:
      | Transform an event into a boolean variable data.
      | - The block transforms every event into a pulse signal with pulse width equal to adopted step size.
      | - Could be used for validation purpose.
      mask Display:
      | disp('')
      | patch([0.88 0.93 0.94 0.99 0.98 0.94 0.9 0.88], [0.11 0.01 0.01 0.11 0.11 0.026 0.11 0.11], [0 1 0])
  LessThan : RelationalOperator  Operator=<  OutDataTypeStr=boolean  ZeroCross=off  RndMeth=Nearest  InputSameDT=on
  Max : MinMax  RequirementInfo={} %GIDa_c2134b07_0c1e_4476_bef8_61dde35be2b3  Function=max  Inputs=2  OutDataTypeStr=Inherit: Inherit via back propagation  SaturateOnIntegerOverflow=on
  Min : MinMax  RequirementInfo={} %GIDa_63ec6bd0_16a7_434f_83f5_af6b3a81d559  Inputs=2  OutDataTypeStr=Inherit: Inherit via back propagation  SaturateOnIntegerOverflow=on
  ScribeInfo : Subsystem  Description=|  mask{BlockComment=|, BlockHistory=|, CommentSeparator=------------, LocalDescription=Description goes here.}
      | Description goes here.
      | ------------
      | Added on : 30-Oct-2015                                                                                                                                               
      | Comments goes there                                                                                                                                                  
      | ------------------------------------                                                                                                                                 
      | Added on : 30-Oct-2015                                                                                                                                               
      | Please keep the dash line as separator,                                                                                                                              
      | last comment is displayed on the mask.                                                                                                                               
      | ------------------------------------
      mask BlockComment=|
      | Added on : 30-Oct-2015
      | Comments goes there
      mask BlockHistory=|
      | Added on : 30-Oct-2015
      | Comments goes there
      | ------------------------------------
      | Added on : 30-Oct-2015
      | Please keep the dash line as separator,
      | last comment is displayed on the mask.
      | ------------------------------------
      mask help:
      | Mask created for improving commenting in model development.
      | v1.0 : creation on november, 2nd 2015
      mask init:
      | % Initialize mask dialog box :
      | % Get the mask handle
      | maskObj          = Simulink.Mask.get(gcb);
      | LocalDescription = get_param(gcb,'LocalDescription');
      | BlockHistory     = get_param(gcb,'BlockHistory');
      | % Set description
      | [Control, ~]   = maskObj.getDialogControl('DescContent');
      | Control.Prompt = LocalDescription;
      | % Set history
      | [Control, ~]   = maskObj.getDialogControl('HistContent');
      | Control.Prompt = BlockHistory;
      mask Display:
      | DescrToPrint = get_param(gcb,'LocalDescription');
      | DescrToPrint = strrep(DescrToPrint,sprintf('\r'),sprintf('\n     '));
      | DescrToPrint = sprintf('Description :\n     %s\n',DescrToPrint);
      | 
      | LastCommentToPrint = get_param(gcb,'BlockComment');
      | LastCommentToPrint = strrep(LastCommentToPrint,sprintf('\r'),sprintf('\n     '));
      | LastCommentToPrint = sprintf('Last Change :\n     %s\n',LastCommentToPrint);
      | 
      | FrontPrint = sprintf('%s\n%s',DescrToPrint,LastCommentToPrint);
      | text(.05,.95,FrontPrint,'verticalalignment','top','horizontalalignment','left');
